simulink model "a1q4"  (R2021b)
settings: Solver=ode23t  StartTime=-0.1  StopTime=0.2  RelTol=1e-3
undefined symbols (not defined in the file or in its folder): d_denSim, d_numSim, denSim, numSim
settings Model: Creator=leos  LastModifiedBy=andre

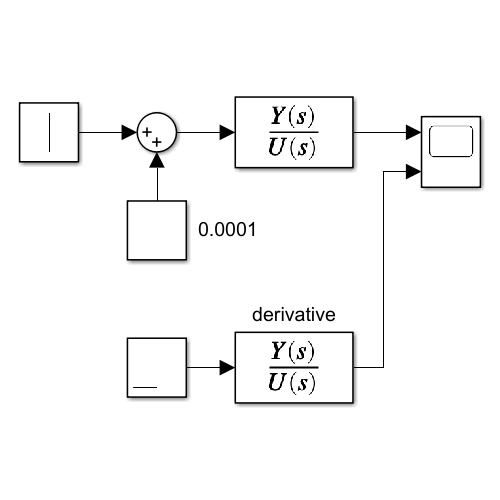
[thumbnail: Simulink's stored preview of the top-level diagram]
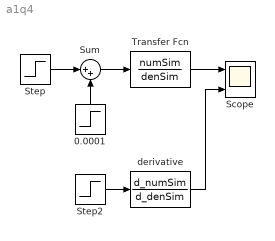
== system a1q4 ==
  0.0001 : Step  Time=0.0001  After=-10000  SampleTime=0
  Scope : Scope  NumInputPorts=2
  Step : Step  Time=0  After=10000  SampleTime=0
  Step2 : Step  Time=0  SampleTime=0
  Sum : Sum  Inputs=|++
  Transfer Fcn : TransferFcn  Numerator=numSim  Denominator=denSim
  derivative : TransferFcn  Numerator=d_numSim  Denominator=d_denSim
  wires:
  Step/1 -> Sum/1
  0.0001/1 -> Sum/2
  Transfer Fcn/1 -> Scope/1
  Sum/1 -> Transfer Fcn/1
  Step2/1 -> derivative/1
  derivative/1 -> Scope/2
